simulink model "8Bit_Processor"  (R2019b)
settings: Solver=FixedStepDiscrete  StartTime=0.0  StopTime=10.0  RelTol=1e-3
libraries: hdlsllib x127, simulink_extras x9
(part 3 of 4)

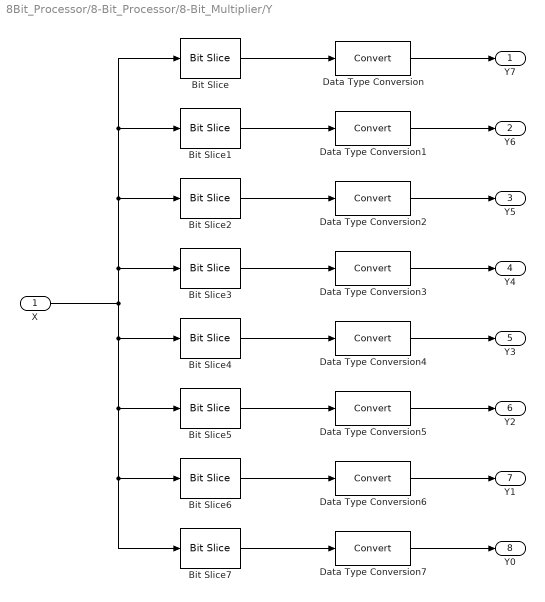
== system 8Bit_Processor/8-Bit_Processor/8-Bit_Multiplier/Y ==
  X : Inport  OutDataTypeStr=uint8  SampleTime=1
  Bit Slice : hdlsllib/Logic and Bit Operations/Bit Slice  lidx=7  ridx=7
      settings: SourceProductName=Simulink  SourceProductBaseCode=SL
  Bit Slice1 : hdlsllib/Logic and Bit Operations/Bit Slice  lidx=6  ridx=6
      settings: SourceProductName=Simulink  SourceProductBaseCode=SL
  Bit Slice2 : hdlsllib/Logic and Bit Operations/Bit Slice  lidx=5  ridx=5
      settings: SourceProductName=Simulink  SourceProductBaseCode=SL
  Bit Slice3 : hdlsllib/Logic and Bit Operations/Bit Slice  lidx=4  ridx=4
      settings: SourceProductName=Simulink  SourceProductBaseCode=SL
  Bit Slice4 : hdlsllib/Logic and Bit Operations/Bit Slice  lidx=3  ridx=3
      settings: SourceProductName=Simulink  SourceProductBaseCode=SL
  Bit Slice5 : hdlsllib/Logic and Bit Operations/Bit Slice  lidx=2  ridx=2
      settings: SourceProductName=Simulink  SourceProductBaseCode=SL
  Bit Slice6 : hdlsllib/Logic and Bit Operations/Bit Slice  lidx=1  ridx=1
      settings: SourceProductName=Simulink  SourceProductBaseCode=SL
  Bit Slice7 : hdlsllib/Logic and Bit Operations/Bit Slice  lidx=0  ridx=0
      settings: SourceProductName=Simulink  SourceProductBaseCode=SL
  Data Type Conversion{,1..7} (8 alike) : DataTypeConversion
  Y7 : Outport
  Y6 : Outport  Port=2
  Y5 : Outport  Port=3
  Y4 : Outport  Port=4
  Y3 : Outport  Port=5
  Y2 : Outport  Port=6
  Y1 : Outport  Port=7
  Y0 : Outport  Port=8
  wires:
  Bit Slice6/1 -> Data Type Conversion6/1
  X/1 -> Bit Slice3/1, Bit Slice2/1, Bit Slice1/1, Bit Slice/1, Bit Slice4/1, Bit Slice5/1, Bit Slice6/1, Bit Slice7/1
  Bit Slice/1 -> Data Type Conversion/1
  Bit Slice7/1 -> Data Type Conversion7/1
  Bit Slice4/1 -> Data Type Conversion4/1
  Bit Slice1/1 -> Data Type Conversion1/1
  Bit Slice3/1 -> Data Type Conversion3/1
  Data Type Conversion1/1 -> Y6/1
  Data Type Conversion7/1 -> Y0/1
  Data Type Conversion5/1 -> Y2/1
  Data Type Conversion3/1 -> Y4/1
  Data Type Conversion4/1 -> Y3/1
  Bit Slice2/1 -> Data Type Conversion2/1
  Bit Slice5/1 -> Data Type Conversion5/1
  Data Type Conversion6/1 -> Y1/1
  Data Type Conversion/1 -> Y7/1
  Data Type Conversion2/1 -> Y5/1

== system 8Bit_Processor/8-Bit_Processor/8-Bit_Register/Concat ==
  X0 : Inport  OutDataTypeStr=boolean  SampleTime=1
  X1 : Inport  Port=2  OutDataTypeStr=boolean  SampleTime=1
  X2 : Inport  Port=3  OutDataTypeStr=boolean  SampleTime=1
  X3 : Inport  Port=4  OutDataTypeStr=boolean  SampleTime=1
  X4 : Inport  Port=5  OutDataTypeStr=boolean  SampleTime=1
  X5 : Inport  Port=6  OutDataTypeStr=boolean  SampleTime=1
  X6 : Inport  Port=7  OutDataTypeStr=boolean  SampleTime=1
  X7 : Inport  Port=8  OutDataTypeStr=boolean  SampleTime=1
  Bit Concat : hdlsllib/Logic and Bit Operations/Bit Concat  numInputs=8
      settings: SourceProductName=Simulink
  Y : Outport  SampleTime=1
  wires:
  X6/1 -> Bit Concat/2
  X2/1 -> Bit Concat/6
  X7/1 -> Bit Concat/1
  X0/1 -> Bit Concat/8
  Bit Concat/1 -> Y/1
  X3/1 -> Bit Concat/5
  X1/1 -> Bit Concat/7
  X5/1 -> Bit Concat/3
  X4/1 -> Bit Concat/4

== system 8Bit_Processor/8-Bit_Processor/8-Bit_Register/Slicer ==
  X : Inport  OutDataTypeStr=uint8  SampleTime=1
  Bit Slice : hdlsllib/Logic and Bit Operations/Bit Slice  lidx=7  ridx=7
      settings: SourceProductName=Simulink  SourceProductBaseCode=SL
  Bit Slice1 : hdlsllib/Logic and Bit Operations/Bit Slice  lidx=6  ridx=6
      settings: SourceProductName=Simulink  SourceProductBaseCode=SL
  Bit Slice2 : hdlsllib/Logic and Bit Operations/Bit Slice  lidx=5  ridx=5
      settings: SourceProductName=Simulink  SourceProductBaseCode=SL
  Bit Slice3 : hdlsllib/Logic and Bit Operations/Bit Slice  lidx=4  ridx=4
      settings: SourceProductName=Simulink  SourceProductBaseCode=SL
  Bit Slice4 : hdlsllib/Logic and Bit Operations/Bit Slice  lidx=3  ridx=3
      settings: SourceProductName=Simulink  SourceProductBaseCode=SL
  Bit Slice5 : hdlsllib/Logic and Bit Operations/Bit Slice  lidx=2  ridx=2
      settings: SourceProductName=Simulink  SourceProductBaseCode=SL
  Bit Slice6 : hdlsllib/Logic and Bit Operations/Bit Slice  lidx=1  ridx=1
      settings: SourceProductName=Simulink  SourceProductBaseCode=SL
  Bit Slice7 : hdlsllib/Logic and Bit Operations/Bit Slice  lidx=0  ridx=0
      settings: SourceProductName=Simulink  SourceProductBaseCode=SL
  Data Type Conversion{,1..7} (8 alike) : DataTypeConversion  OutDataTypeStr=boolean
  Y7 : Outport  OutDataTypeStr=boolean  SampleTime=1
  Y6 : Outport  Port=2  OutDataTypeStr=boolean  SampleTime=1
  Y5 : Outport  Port=3  OutDataTypeStr=boolean  SampleTime=1
  Y4 : Outport  Port=4  OutDataTypeStr=boolean
  Y3 : Outport  Port=5  OutDataTypeStr=boolean  SampleTime=1
  Y2 : Outport  Port=6  OutDataTypeStr=boolean  SampleTime=1
  Y1 : Outport  Port=7  OutDataTypeStr=boolean  SampleTime=1
  Y0 : Outport  Port=8  OutDataTypeStr=boolean  SampleTime=1
  wires:
  Bit Slice6/1 -> Data Type Conversion6/1
  X/1 -> Bit Slice3/1, Bit Slice2/1, Bit Slice1/1, Bit Slice/1, Bit Slice4/1, Bit Slice5/1, Bit Slice6/1, Bit Slice7/1
  Bit Slice/1 -> Data Type Conversion/1
  Bit Slice7/1 -> Data Type Conversion7/1
  Bit Slice4/1 -> Data Type Conversion4/1
  Bit Slice1/1 -> Data Type Conversion1/1
  Bit Slice3/1 -> Data Type Conversion3/1
  Data Type Conversion1/1 -> Y6/1
  Data Type Conversion7/1 -> Y0/1
  Data Type Conversion5/1 -> Y2/1
  Data Type Conversion3/1 -> Y4/1
  Data Type Conversion4/1 -> Y3/1
  Bit Slice2/1 -> Data Type Conversion2/1
  Bit Slice5/1 -> Data Type Conversion5/1
  Data Type Conversion6/1 -> Y1/1
  Data Type Conversion/1 -> Y7/1
  Data Type Conversion2/1 -> Y5/1

== system 8Bit_Processor/8-Bit_Processor/8-Bit_Subtractor/Concat1 ==
  X7 : Inport  OutDataTypeStr=boolean  SampleTime=1
  X6 : Inport  Port=2  OutDataTypeStr=boolean  SampleTime=1
  X5 : Inport  Port=3  OutDataTypeStr=boolean  SampleTime=1
  X4 : Inport  Port=4  OutDataTypeStr=boolean  SampleTime=1
  X3 : Inport  Port=5  OutDataTypeStr=boolean  SampleTime=1
  X2 : Inport  Port=6  OutDataTypeStr=boolean  SampleTime=1
  X1 : Inport  Port=7  OutDataTypeStr=boolean  SampleTime=1
  X0 : Inport  Port=8  OutDataTypeStr=boolean  SampleTime=1
  Bit Concat : hdlsllib/Logic and Bit Operations/Bit Concat  numInputs=8
      settings: SourceProductName=Simulink
  Y : Outport
  wires:
  X6/1 -> Bit Concat/2
  X2/1 -> Bit Concat/6
  X7/1 -> Bit Concat/1
  X0/1 -> Bit Concat/8
  Bit Concat/1 -> Y/1
  X3/1 -> Bit Concat/5
  X1/1 -> Bit Concat/7
  X5/1 -> Bit Concat/3
  X4/1 -> Bit Concat/4

== system 8Bit_Processor/8-Bit_Processor/8-Bit_Subtractor/Full Subtractor ==
  In1 : Inport  OutDataTypeStr=boolean
  In2 : Inport  Port=2  OutDataTypeStr=boolean
  In3 : Inport  Port=3  OutDataTypeStr=boolean
  Half subtractor : Subsystem
  Half subtractor1 : Subsystem
  Logical Operator1 : Logic  Operator=OR  AllPortsSameDT=off  OutDataTypeStr=boolean
  Out1 : Outport
  Out2 : Outport  Port=2
  wires:
  Logical Operator1/1 -> Out2/1
  In1/1 -> Half subtractor/1(In1)
  Half subtractor1/1(Out1) -> Out1/1
  In2/1 -> Half subtractor/2(In2)
  In3/1 -> Half subtractor1/2(In2)
  Half subtractor/2(Out2) -> Logical Operator1/2
  Half subtractor/1(Out1) -> Half subtractor1/1(In1)
  Half subtractor1/2(Out2) -> Logical Operator1/1

== system 8Bit_Processor/8-Bit_Processor/8-Bit_Subtractor/Full Subtractor 2 ==
  In1 : Inport  OutDataTypeStr=boolean
  In2 : Inport  Port=2  OutDataTypeStr=boolean
  In3 : Inport  Port=3  OutDataTypeStr=boolean
  Half subtractor : Subsystem
  Half subtractor1 : Subsystem
  Logical Operator1 : Logic  Operator=OR  AllPortsSameDT=off  OutDataTypeStr=boolean
  Out1 : Outport
  Out2 : Outport  Port=2
  wires:
  Logical Operator1/1 -> Out2/1
  In1/1 -> Half subtractor/1(In1)
  Half subtractor1/1(Out1) -> Out1/1
  In2/1 -> Half subtractor/2(In2)
  In3/1 -> Half subtractor1/2(In2)
  Half subtractor/2(Out2) -> Logical Operator1/2
  Half subtractor/1(Out1) -> Half subtractor1/1(In1)
  Half subtractor1/2(Out2) -> Logical Operator1/1

== system 8Bit_Processor/8-Bit_Processor/8-Bit_Subtractor/Full Subtractor 3 ==
  In1 : Inport  OutDataTypeStr=boolean
  In2 : Inport  Port=2  OutDataTypeStr=boolean
  In3 : Inport  Port=3  OutDataTypeStr=boolean
  Half subtractor : Subsystem
  Half subtractor1 : Subsystem
  Logical Operator1 : Logic  Operator=OR  AllPortsSameDT=off  OutDataTypeStr=boolean
  Out1 : Outport
  Out2 : Outport  Port=2
  wires:
  Logical Operator1/1 -> Out2/1
  In1/1 -> Half subtractor/1(In1)
  Half subtractor1/1(Out1) -> Out1/1
  In2/1 -> Half subtractor/2(In2)
  In3/1 -> Half subtractor1/2(In2)
  Half subtractor/2(Out2) -> Logical Operator1/2
  Half subtractor/1(Out1) -> Half subtractor1/1(In1)
  Half subtractor1/2(Out2) -> Logical Operator1/1

== system 8Bit_Processor/8-Bit_Processor/8-Bit_Subtractor/Full Subtractor 4 ==
  In1 : Inport  OutDataTypeStr=boolean
  In2 : Inport  Port=2  OutDataTypeStr=boolean
  In3 : Inport  Port=3  OutDataTypeStr=boolean
  Half subtractor : Subsystem
  Half subtractor1 : Subsystem
  Logical Operator1 : Logic  Operator=OR  AllPortsSameDT=off  OutDataTypeStr=boolean
  Out1 : Outport
  Out2 : Outport  Port=2
  wires:
  Logical Operator1/1 -> Out2/1
  In1/1 -> Half subtractor/1(In1)
  Half subtractor1/1(Out1) -> Out1/1
  In2/1 -> Half subtractor/2(In2)
  In3/1 -> Half subtractor1/2(In2)
  Half subtractor/2(Out2) -> Logical Operator1/2
  Half subtractor/1(Out1) -> Half subtractor1/1(In1)
  Half subtractor1/2(Out2) -> Logical Operator1/1

== system 8Bit_Processor/8-Bit_Processor/8-Bit_Subtractor/Full Subtractor 5 ==
  In1 : Inport  OutDataTypeStr=boolean
  In2 : Inport  Port=2  OutDataTypeStr=boolean
  In3 : Inport  Port=3  OutDataTypeStr=boolean
  Half subtractor : Subsystem
  Half subtractor1 : Subsystem
  Logical Operator1 : Logic  Operator=OR  AllPortsSameDT=off  OutDataTypeStr=boolean
  Out1 : Outport
  Out2 : Outport  Port=2
  wires:
  Logical Operator1/1 -> Out2/1
  In1/1 -> Half subtractor/1(In1)
  Half subtractor1/1(Out1) -> Out1/1
  In2/1 -> Half subtractor/2(In2)
  In3/1 -> Half subtractor1/2(In2)
  Half subtractor/2(Out2) -> Logical Operator1/2
  Half subtractor/1(Out1) -> Half subtractor1/1(In1)
  Half subtractor1/2(Out2) -> Logical Operator1/1

== system 8Bit_Processor/8-Bit_Processor/8-Bit_Subtractor/Full Subtractor 6 ==
  In1 : Inport  OutDataTypeStr=boolean
  In2 : Inport  Port=2  OutDataTypeStr=boolean
  In3 : Inport  Port=3  OutDataTypeStr=boolean
  Half subtractor : Subsystem
  Half subtractor1 : Subsystem
  Logical Operator1 : Logic  Operator=OR  AllPortsSameDT=off  OutDataTypeStr=boolean
  Out1 : Outport
  Out2 : Outport  Port=2
  wires:
  Logical Operator1/1 -> Out2/1
  In1/1 -> Half subtractor/1(In1)
  Half subtractor1/1(Out1) -> Out1/1
  In2/1 -> Half subtractor/2(In2)
  In3/1 -> Half subtractor1/2(In2)
  Half subtractor/2(Out2) -> Logical Operator1/2
  Half subtractor/1(Out1) -> Half subtractor1/1(In1)
  Half subtractor1/2(Out2) -> Logical Operator1/1

== system 8Bit_Processor/8-Bit_Processor/8-Bit_Subtractor/Full Subtractor 7 ==
  In1 : Inport  OutDataTypeStr=boolean
  In2 : Inport  Port=2  OutDataTypeStr=boolean
  In3 : Inport  Port=3  OutDataTypeStr=boolean
  Half subtractor : Subsystem
  Half subtractor1 : Subsystem
  Logical Operator1 : Logic  Operator=OR  AllPortsSameDT=off  OutDataTypeStr=boolean
  Out1 : Outport
  Out2 : Outport  Port=2
  wires:
  Logical Operator1/1 -> Out2/1
  In1/1 -> Half subtractor/1(In1)
  Half subtractor1/1(Out1) -> Out1/1
  In2/1 -> Half subtractor/2(In2)
  In3/1 -> Half subtractor1/2(In2)
  Half subtractor/2(Out2) -> Logical Operator1/2
  Half subtractor/1(Out1) -> Half subtractor1/1(In1)
  Half subtractor1/2(Out2) -> Logical Operator1/1

== system 8Bit_Processor/8-Bit_Processor/8-Bit_Subtractor/Half subtractor ==
  In1 : Inport  OutDataTypeStr=boolean
  In2 : Inport  Port=2  OutDataTypeStr=boolean
  Logical Operator : Logic  AllPortsSameDT=off  OutDataTypeStr=boolean
  Logical Operator1 : Logic  Operator=XOR  AllPortsSameDT=off  OutDataTypeStr=boolean
  NOT : Logic  Operator=NOT  IconShape=distinctive  AllPortsSameDT=off  OutDataTypeStr=boolean
  Out1 : Outport
  Out2 : Outport  Port=2
  wires:
  In2/1 -> Logical Operator/2, Logical Operator1/2
  In1/1 -> NOT/1, Logical Operator1/1
  Logical Operator1/1 -> Out1/1
  Logical Operator/1 -> Out2/1
  NOT/1 -> Logical Operator/1

== system 8Bit_Processor/8-Bit_Processor/8-Bit_Subtractor/Slicer1 ==
  X : Inport  OutDataTypeStr=uint8  SampleTime=1
  Bit Slice : hdlsllib/Logic and Bit Operations/Bit Slice  lidx=7  ridx=7
      settings: SourceProductName=Simulink  SourceProductBaseCode=SL
  Bit Slice1 : hdlsllib/Logic and Bit Operations/Bit Slice  lidx=6  ridx=6
      settings: SourceProductName=Simulink  SourceProductBaseCode=SL
  Bit Slice2 : hdlsllib/Logic and Bit Operations/Bit Slice  lidx=5  ridx=5
      settings: SourceProductName=Simulink  SourceProductBaseCode=SL
  Bit Slice3 : hdlsllib/Logic and Bit Operations/Bit Slice  lidx=4  ridx=4
      settings: SourceProductName=Simulink  SourceProductBaseCode=SL
  Bit Slice4 : hdlsllib/Logic and Bit Operations/Bit Slice  lidx=3  ridx=3
      settings: SourceProductName=Simulink  SourceProductBaseCode=SL
  Bit Slice5 : hdlsllib/Logic and Bit Operations/Bit Slice  lidx=2  ridx=2
      settings: SourceProductName=Simulink  SourceProductBaseCode=SL
  Bit Slice6 : hdlsllib/Logic and Bit Operations/Bit Slice  lidx=1  ridx=1
      settings: SourceProductName=Simulink  SourceProductBaseCode=SL
  Bit Slice7 : hdlsllib/Logic and Bit Operations/Bit Slice  lidx=0  ridx=0
      settings: SourceProductName=Simulink  SourceProductBaseCode=SL
  Data Type Conversion{,1..7} (8 alike) : DataTypeConversion
  Y7 : Outport
  Y6 : Outport  Port=2
  Y5 : Outport  Port=3
  Y4 : Outport  Port=4
  Y3 : Outport  Port=5
  Y2 : Outport  Port=6
  Y1 : Outport  Port=7
  Y0 : Outport  Port=8
  wires:
  Bit Slice6/1 -> Data Type Conversion6/1
  X/1 -> Bit Slice3/1, Bit Slice2/1, Bit Slice1/1, Bit Slice/1, Bit Slice4/1, Bit Slice5/1, Bit Slice6/1, Bit Slice7/1
  Bit Slice/1 -> Data Type Conversion/1
  Bit Slice7/1 -> Data Type Conversion7/1
  Bit Slice4/1 -> Data Type Conversion4/1
  Bit Slice1/1 -> Data Type Conversion1/1
  Bit Slice3/1 -> Data Type Conversion3/1
  Data Type Conversion1/1 -> Y6/1
  Data Type Conversion7/1 -> Y0/1
  Data Type Conversion5/1 -> Y2/1
  Data Type Conversion3/1 -> Y4/1
  Data Type Conversion4/1 -> Y3/1
  Bit Slice2/1 -> Data Type Conversion2/1
  Bit Slice5/1 -> Data Type Conversion5/1
  Data Type Conversion6/1 -> Y1/1
  Data Type Conversion/1 -> Y7/1
  Data Type Conversion2/1 -> Y5/1

== system 8Bit_Processor/8-Bit_Processor/8-Bit_Subtractor/Slicer2 ==
  X : Inport  OutDataTypeStr=uint8  SampleTime=1
  Bit Slice : hdlsllib/Logic and Bit Operations/Bit Slice  lidx=7  ridx=7
      settings: SourceProductName=Simulink  SourceProductBaseCode=SL
  Bit Slice1 : hdlsllib/Logic and Bit Operations/Bit Slice  lidx=6  ridx=6
      settings: SourceProductName=Simulink  SourceProductBaseCode=SL
  Bit Slice2 : hdlsllib/Logic and Bit Operations/Bit Slice  lidx=5  ridx=5
      settings: SourceProductName=Simulink  SourceProductBaseCode=SL
  Bit Slice3 : hdlsllib/Logic and Bit Operations/Bit Slice  lidx=4  ridx=4
      settings: SourceProductName=Simulink  SourceProductBaseCode=SL
  Bit Slice4 : hdlsllib/Logic and Bit Operations/Bit Slice  lidx=3  ridx=3
      settings: SourceProductName=Simulink  SourceProductBaseCode=SL
  Bit Slice5 : hdlsllib/Logic and Bit Operations/Bit Slice  lidx=2  ridx=2
      settings: SourceProductName=Simulink  SourceProductBaseCode=SL
  Bit Slice6 : hdlsllib/Logic and Bit Operations/Bit Slice  lidx=1  ridx=1
      settings: SourceProductName=Simulink  SourceProductBaseCode=SL
  Bit Slice7 : hdlsllib/Logic and Bit Operations/Bit Slice  lidx=0  ridx=0
      settings: SourceProductName=Simulink  SourceProductBaseCode=SL
  Data Type Conversion{,1..7} (8 alike) : DataTypeConversion
  Y7 : Outport
  Y6 : Outport  Port=2
  Y5 : Outport  Port=3
  Y4 : Outport  Port=4
  Y3 : Outport  Port=5
  Y2 : Outport  Port=6
  Y1 : Outport  Port=7
  Y0 : Outport  Port=8
  wires:
  Bit Slice6/1 -> Data Type Conversion6/1
  X/1 -> Bit Slice3/1, Bit Slice2/1, Bit Slice1/1, Bit Slice/1, Bit Slice4/1, Bit Slice5/1, Bit Slice6/1, Bit Slice7/1
  Bit Slice/1 -> Data Type Conversion/1
  Bit Slice7/1 -> Data Type Conversion7/1
  Bit Slice4/1 -> Data Type Conversion4/1
  Bit Slice1/1 -> Data Type Conversion1/1
  Bit Slice3/1 -> Data Type Conversion3/1
  Data Type Conversion1/1 -> Y6/1
  Data Type Conversion7/1 -> Y0/1
  Data Type Conversion5/1 -> Y2/1
  Data Type Conversion3/1 -> Y4/1
  Data Type Conversion4/1 -> Y3/1
  Bit Slice2/1 -> Data Type Conversion2/1
  Bit Slice5/1 -> Data Type Conversion5/1
  Data Type Conversion6/1 -> Y1/1
  Data Type Conversion/1 -> Y7/1
  Data Type Conversion2/1 -> Y5/1

== system 8Bit_Processor/8-Bit_Processor/8-Bit 4-to-1 MUX/Subsystem/Slicer ==
  X : Inport  SampleTime=1
  Bit Slice6 : hdlsllib/Logic and Bit Operations/Bit Slice  lidx=1  ridx=1
      settings: SourceProductName=Simulink  SourceProductBaseCode=SL
  Bit Slice7 : hdlsllib/Logic and Bit Operations/Bit Slice  lidx=0  ridx=0
      settings: SourceProductName=Simulink  SourceProductBaseCode=SL
  Data Type Conversion6 : DataTypeConversion  OutDataTypeStr=boolean
  Data Type Conversion7 : DataTypeConversion  OutDataTypeStr=boolean
  A : Outport  OutDataTypeStr=boolean  SampleTime=1
  B : Outport  Port=2  OutDataTypeStr=boolean  SampleTime=1
  wires:
  Bit Slice6/1 -> Data Type Conversion6/1
  X/1 -> Bit Slice6/1, Bit Slice7/1
  Bit Slice7/1 -> Data Type Conversion7/1
  Data Type Conversion7/1 -> A/1
  Data Type Conversion6/1 -> B/1

== system 8Bit_Processor/8-Bit_Processor/8-Bit 4-to-1 MUX/Subsystem1/Slicer ==
  X : Inport  SampleTime=1
  Bit Slice6 : hdlsllib/Logic and Bit Operations/Bit Slice  lidx=1  ridx=1
      settings: SourceProductName=Simulink  SourceProductBaseCode=SL
  Bit Slice7 : hdlsllib/Logic and Bit Operations/Bit Slice  lidx=0  ridx=0
      settings: SourceProductName=Simulink  SourceProductBaseCode=SL
  Data Type Conversion6 : DataTypeConversion  OutDataTypeStr=boolean
  Data Type Conversion7 : DataTypeConversion  OutDataTypeStr=boolean
  A : Outport  OutDataTypeStr=boolean  SampleTime=1
  B : Outport  Port=2  OutDataTypeStr=boolean  SampleTime=1
  wires:
  Bit Slice6/1 -> Data Type Conversion6/1
  X/1 -> Bit Slice6/1, Bit Slice7/1
  Bit Slice7/1 -> Data Type Conversion7/1
  Data Type Conversion7/1 -> A/1
  Data Type Conversion6/1 -> B/1

== system 8Bit_Processor/8-Bit_Processor/8-Bit 4-to-1 MUX/Subsystem2/Slicer ==
  X : Inport  SampleTime=1
  Bit Slice6 : hdlsllib/Logic and Bit Operations/Bit Slice  lidx=1  ridx=1
      settings: SourceProductName=Simulink  SourceProductBaseCode=SL
  Bit Slice7 : hdlsllib/Logic and Bit Operations/Bit Slice  lidx=0  ridx=0
      settings: SourceProductName=Simulink  SourceProductBaseCode=SL
  Data Type Conversion6 : DataTypeConversion  OutDataTypeStr=boolean
  Data Type Conversion7 : DataTypeConversion  OutDataTypeStr=boolean
  A : Outport  OutDataTypeStr=boolean  SampleTime=1
  B : Outport  Port=2  OutDataTypeStr=boolean  SampleTime=1
  wires:
  Bit Slice6/1 -> Data Type Conversion6/1
  X/1 -> Bit Slice6/1, Bit Slice7/1
  Bit Slice7/1 -> Data Type Conversion7/1
  Data Type Conversion7/1 -> A/1
  Data Type Conversion6/1 -> B/1

== system 8Bit_Processor/8-Bit_Processor/8-Bit 4-to-1 MUX/Subsystem3/Slicer ==
  X : Inport  SampleTime=1
  Bit Slice6 : hdlsllib/Logic and Bit Operations/Bit Slice  lidx=1  ridx=1
      settings: SourceProductName=Simulink  SourceProductBaseCode=SL
  Bit Slice7 : hdlsllib/Logic and Bit Operations/Bit Slice  lidx=0  ridx=0
      settings: SourceProductName=Simulink  SourceProductBaseCode=SL
  Data Type Conversion6 : DataTypeConversion  OutDataTypeStr=boolean
  Data Type Conversion7 : DataTypeConversion  OutDataTypeStr=boolean
  A : Outport  OutDataTypeStr=boolean  SampleTime=1
  B : Outport  Port=2  OutDataTypeStr=boolean  SampleTime=1
  wires:
  Bit Slice6/1 -> Data Type Conversion6/1
  X/1 -> Bit Slice6/1, Bit Slice7/1
  Bit Slice7/1 -> Data Type Conversion7/1
  Data Type Conversion7/1 -> A/1
  Data Type Conversion6/1 -> B/1

== system 8Bit_Processor/8-Bit_Processor/8-Bit 4-to-1 MUX/Subsystem4/Slicer ==
  X : Inport  SampleTime=1
  Bit Slice6 : hdlsllib/Logic and Bit Operations/Bit Slice  lidx=1  ridx=1
      settings: SourceProductName=Simulink  SourceProductBaseCode=SL
  Bit Slice7 : hdlsllib/Logic and Bit Operations/Bit Slice  lidx=0  ridx=0
      settings: SourceProductName=Simulink  SourceProductBaseCode=SL
  Data Type Conversion6 : DataTypeConversion  OutDataTypeStr=boolean
  Data Type Conversion7 : DataTypeConversion  OutDataTypeStr=boolean
  A : Outport  OutDataTypeStr=boolean  SampleTime=1
  B : Outport  Port=2  OutDataTypeStr=boolean  SampleTime=1
  wires:
  Bit Slice6/1 -> Data Type Conversion6/1
  X/1 -> Bit Slice6/1, Bit Slice7/1
  Bit Slice7/1 -> Data Type Conversion7/1
  Data Type Conversion7/1 -> A/1
  Data Type Conversion6/1 -> B/1

== system 8Bit_Processor/8-Bit_Processor/8-Bit 4-to-1 MUX/Subsystem5/Slicer ==
  X : Inport  SampleTime=1
  Bit Slice6 : hdlsllib/Logic and Bit Operations/Bit Slice  lidx=1  ridx=1
      settings: SourceProductName=Simulink  SourceProductBaseCode=SL
  Bit Slice7 : hdlsllib/Logic and Bit Operations/Bit Slice  lidx=0  ridx=0
      settings: SourceProductName=Simulink  SourceProductBaseCode=SL
  Data Type Conversion6 : DataTypeConversion  OutDataTypeStr=boolean
  Data Type Conversion7 : DataTypeConversion  OutDataTypeStr=boolean
  A : Outport  OutDataTypeStr=boolean  SampleTime=1
  B : Outport  Port=2  OutDataTypeStr=boolean  SampleTime=1
  wires:
  Bit Slice6/1 -> Data Type Conversion6/1
  X/1 -> Bit Slice6/1, Bit Slice7/1
  Bit Slice7/1 -> Data Type Conversion7/1
  Data Type Conversion7/1 -> A/1
  Data Type Conversion6/1 -> B/1

== system 8Bit_Processor/8-Bit_Processor/8-Bit 4-to-1 MUX/Subsystem6/Slicer ==
  X : Inport  SampleTime=1
  Bit Slice6 : hdlsllib/Logic and Bit Operations/Bit Slice  lidx=1  ridx=1
      settings: SourceProductName=Simulink  SourceProductBaseCode=SL
  Bit Slice7 : hdlsllib/Logic and Bit Operations/Bit Slice  lidx=0  ridx=0
      settings: SourceProductName=Simulink  SourceProductBaseCode=SL
  Data Type Conversion6 : DataTypeConversion  OutDataTypeStr=boolean
  Data Type Conversion7 : DataTypeConversion  OutDataTypeStr=boolean
  A : Outport  OutDataTypeStr=boolean  SampleTime=1
  B : Outport  Port=2  OutDataTypeStr=boolean  SampleTime=1
  wires:
  Bit Slice6/1 -> Data Type Conversion6/1
  X/1 -> Bit Slice6/1, Bit Slice7/1
  Bit Slice7/1 -> Data Type Conversion7/1
  Data Type Conversion7/1 -> A/1
  Data Type Conversion6/1 -> B/1

== system 8Bit_Processor/8-Bit_Processor/8-Bit 4-to-1 MUX/Subsystem7/Slicer ==
  X : Inport  SampleTime=1
  Bit Slice6 : hdlsllib/Logic and Bit Operations/Bit Slice  lidx=1  ridx=1
      settings: SourceProductName=Simulink  SourceProductBaseCode=SL
  Bit Slice7 : hdlsllib/Logic and Bit Operations/Bit Slice  lidx=0  ridx=0
      settings: SourceProductName=Simulink  SourceProductBaseCode=SL
  Data Type Conversion6 : DataTypeConversion  OutDataTypeStr=boolean
  Data Type Conversion7 : DataTypeConversion  OutDataTypeStr=boolean
  A : Outport  OutDataTypeStr=boolean  SampleTime=1
  B : Outport  Port=2  OutDataTypeStr=boolean  SampleTime=1
  wires:
  Bit Slice6/1 -> Data Type Conversion6/1
  X/1 -> Bit Slice6/1, Bit Slice7/1
  Bit Slice7/1 -> Data Type Conversion7/1
  Data Type Conversion7/1 -> A/1
  Data Type Conversion6/1 -> B/1

== system 8Bit_Processor/8-Bit_Processor/8-Bit_Adder/Full adder1/Half adder1 ==
  In1 : Inport  OutDataTypeStr=boolean
  In2 : Inport  Port=2  OutDataTypeStr=boolean
  Logical Operator : Logic  AllPortsSameDT=off  OutDataTypeStr=boolean
  Logical Operator1 : Logic  Operator=XOR  AllPortsSameDT=off  OutDataTypeStr=boolean
  Out1 : Outport
  Out2 : Outport  Port=2
  wires:
  In2/1 -> Logical Operator/2, Logical Operator1/2
  In1/1 -> Logical Operator/1, Logical Operator1/1
  Logical Operator1/1 -> Out1/1
  Logical Operator/1 -> Out2/1

== system 8Bit_Processor/8-Bit_Processor/8-Bit_Adder/Full adder1/Half adder2 ==
  In1 : Inport  OutDataTypeStr=boolean
  In2 : Inport  Port=2  OutDataTypeStr=boolean
  Logical Operator : Logic  AllPortsSameDT=off  OutDataTypeStr=boolean
  Logical Operator1 : Logic  Operator=XOR  AllPortsSameDT=off  OutDataTypeStr=boolean
  Out1 : Outport
  Out2 : Outport  Port=2
  wires:
  In2/1 -> Logical Operator/2, Logical Operator1/2
  In1/1 -> Logical Operator/1, Logical Operator1/1
  Logical Operator1/1 -> Out1/1
  Logical Operator/1 -> Out2/1

== system 8Bit_Processor/8-Bit_Processor/8-Bit_Adder/Full adder2/Half adder1 ==
  In1 : Inport  OutDataTypeStr=boolean
  In2 : Inport  Port=2  OutDataTypeStr=boolean
  Logical Operator : Logic  AllPortsSameDT=off  OutDataTypeStr=boolean
  Logical Operator1 : Logic  Operator=XOR  AllPortsSameDT=off  OutDataTypeStr=boolean
  Out1 : Outport
  Out2 : Outport  Port=2
  wires:
  In2/1 -> Logical Operator/2, Logical Operator1/2
  In1/1 -> Logical Operator/1, Logical Operator1/1
  Logical Operator1/1 -> Out1/1
  Logical Operator/1 -> Out2/1

== system 8Bit_Processor/8-Bit_Processor/8-Bit_Adder/Full adder2/Half adder2 ==
  In1 : Inport  OutDataTypeStr=boolean
  In2 : Inport  Port=2  OutDataTypeStr=boolean
  Logical Operator : Logic  AllPortsSameDT=off  OutDataTypeStr=boolean
  Logical Operator1 : Logic  Operator=XOR  AllPortsSameDT=off  OutDataTypeStr=boolean
  Out1 : Outport
  Out2 : Outport  Port=2
  wires:
  In2/1 -> Logical Operator/2, Logical Operator1/2
  In1/1 -> Logical Operator/1, Logical Operator1/1
  Logical Operator1/1 -> Out1/1
  Logical Operator/1 -> Out2/1

== system 8Bit_Processor/8-Bit_Processor/8-Bit_Adder/Full adder3/Half adder1 ==
  In1 : Inport  OutDataTypeStr=boolean
  In2 : Inport  Port=2  OutDataTypeStr=boolean
  Logical Operator : Logic  AllPortsSameDT=off  OutDataTypeStr=boolean
  Logical Operator1 : Logic  Operator=XOR  AllPortsSameDT=off  OutDataTypeStr=boolean
  Out1 : Outport
  Out2 : Outport  Port=2
  wires:
  In2/1 -> Logical Operator/2, Logical Operator1/2
  In1/1 -> Logical Operator/1, Logical Operator1/1
  Logical Operator1/1 -> Out1/1
  Logical Operator/1 -> Out2/1

== system 8Bit_Processor/8-Bit_Processor/8-Bit_Adder/Full adder3/Half adder2 ==
  In1 : Inport  OutDataTypeStr=boolean
  In2 : Inport  Port=2  OutDataTypeStr=boolean
  Logical Operator : Logic  AllPortsSameDT=off  OutDataTypeStr=boolean
  Logical Operator1 : Logic  Operator=XOR  AllPortsSameDT=off  OutDataTypeStr=boolean
  Out1 : Outport
  Out2 : Outport  Port=2
  wires:
  In2/1 -> Logical Operator/2, Logical Operator1/2
  In1/1 -> Logical Operator/1, Logical Operator1/1
  Logical Operator1/1 -> Out1/1
  Logical Operator/1 -> Out2/1

== system 8Bit_Processor/8-Bit_Processor/8-Bit_Adder/Full adder4/Half adder1 ==
  In1 : Inport  OutDataTypeStr=boolean
  In2 : Inport  Port=2  OutDataTypeStr=boolean
  Logical Operator : Logic  AllPortsSameDT=off  OutDataTypeStr=boolean
  Logical Operator1 : Logic  Operator=XOR  AllPortsSameDT=off  OutDataTypeStr=boolean
  Out1 : Outport
  Out2 : Outport  Port=2
  wires:
  In2/1 -> Logical Operator/2, Logical Operator1/2
  In1/1 -> Logical Operator/1, Logical Operator1/1
  Logical Operator1/1 -> Out1/1
  Logical Operator/1 -> Out2/1

== system 8Bit_Processor/8-Bit_Processor/8-Bit_Adder/Full adder4/Half adder2 ==
  In1 : Inport  OutDataTypeStr=boolean
  In2 : Inport  Port=2  OutDataTypeStr=boolean
  Logical Operator : Logic  AllPortsSameDT=off  OutDataTypeStr=boolean
  Logical Operator1 : Logic  Operator=XOR  AllPortsSameDT=off  OutDataTypeStr=boolean
  Out1 : Outport
  Out2 : Outport  Port=2
  wires:
  In2/1 -> Logical Operator/2, Logical Operator1/2
  In1/1 -> Logical Operator/1, Logical Operator1/1
  Logical Operator1/1 -> Out1/1
  Logical Operator/1 -> Out2/1

== system 8Bit_Processor/8-Bit_Processor/8-Bit_Adder/Full adder5/Half adder1 ==
  In1 : Inport  OutDataTypeStr=boolean
  In2 : Inport  Port=2  OutDataTypeStr=boolean
  Logical Operator : Logic  AllPortsSameDT=off  OutDataTypeStr=boolean
  Logical Operator1 : Logic  Operator=XOR  AllPortsSameDT=off  OutDataTypeStr=boolean
  Out1 : Outport
  Out2 : Outport  Port=2
  wires:
  In2/1 -> Logical Operator/2, Logical Operator1/2
  In1/1 -> Logical Operator/1, Logical Operator1/1
  Logical Operator1/1 -> Out1/1
  Logical Operator/1 -> Out2/1

== system 8Bit_Processor/8-Bit_Processor/8-Bit_Adder/Full adder5/Half adder2 ==
  In1 : Inport  OutDataTypeStr=boolean
  In2 : Inport  Port=2  OutDataTypeStr=boolean
  Logical Operator : Logic  AllPortsSameDT=off  OutDataTypeStr=boolean
  Logical Operator1 : Logic  Operator=XOR  AllPortsSameDT=off  OutDataTypeStr=boolean
  Out1 : Outport
  Out2 : Outport  Port=2
  wires:
  In2/1 -> Logical Operator/2, Logical Operator1/2
  In1/1 -> Logical Operator/1, Logical Operator1/1
  Logical Operator1/1 -> Out1/1
  Logical Operator/1 -> Out2/1

== system 8Bit_Processor/8-Bit_Processor/8-Bit_Adder/Full adder6/Half adder1 ==
  In1 : Inport  OutDataTypeStr=boolean
  In2 : Inport  Port=2  OutDataTypeStr=boolean
  Logical Operator : Logic  AllPortsSameDT=off  OutDataTypeStr=boolean
  Logical Operator1 : Logic  Operator=XOR  AllPortsSameDT=off  OutDataTypeStr=boolean
  Out1 : Outport
  Out2 : Outport  Port=2
  wires:
  In2/1 -> Logical Operator/2, Logical Operator1/2
  In1/1 -> Logical Operator/1, Logical Operator1/1
  Logical Operator1/1 -> Out1/1
  Logical Operator/1 -> Out2/1

== system 8Bit_Processor/8-Bit_Processor/8-Bit_Adder/Full adder6/Half adder2 ==
  In1 : Inport  OutDataTypeStr=boolean
  In2 : Inport  Port=2  OutDataTypeStr=boolean
  Logical Operator : Logic  AllPortsSameDT=off  OutDataTypeStr=boolean
  Logical Operator1 : Logic  Operator=XOR  AllPortsSameDT=off  OutDataTypeStr=boolean
  Out1 : Outport
  Out2 : Outport  Port=2
  wires:
  In2/1 -> Logical Operator/2, Logical Operator1/2
  In1/1 -> Logical Operator/1, Logical Operator1/1
  Logical Operator1/1 -> Out1/1
  Logical Operator/1 -> Out2/1

== system 8Bit_Processor/8-Bit_Processor/8-Bit_Adder/Full adder7/Half adder1 ==
  In1 : Inport  OutDataTypeStr=boolean
  In2 : Inport  Port=2  OutDataTypeStr=boolean
  Logical Operator : Logic  AllPortsSameDT=off  OutDataTypeStr=boolean
  Logical Operator1 : Logic  Operator=XOR  AllPortsSameDT=off  OutDataTypeStr=boolean
  Out1 : Outport
  Out2 : Outport  Port=2
  wires:
  In2/1 -> Logical Operator/2, Logical Operator1/2
  In1/1 -> Logical Operator/1, Logical Operator1/1
  Logical Operator1/1 -> Out1/1
  Logical Operator/1 -> Out2/1

== system 8Bit_Processor/8-Bit_Processor/8-Bit_Adder/Full adder7/Half adder2 ==
  In1 : Inport  OutDataTypeStr=boolean
  In2 : Inport  Port=2  OutDataTypeStr=boolean
  Logical Operator : Logic  AllPortsSameDT=off  OutDataTypeStr=boolean
  Logical Operator1 : Logic  Operator=XOR  AllPortsSameDT=off  OutDataTypeStr=boolean
  Out1 : Outport
  Out2 : Outport  Port=2
  wires:
  In2/1 -> Logical Operator/2, Logical Operator1/2
  In1/1 -> Logical Operator/1, Logical Operator1/1
  Logical Operator1/1 -> Out1/1
  Logical Operator/1 -> Out2/1

== system 8Bit_Processor/8-Bit_Processor/8-Bit_Multiplier/Full adder1/Half adder1 ==
  In1 : Inport  OutDataTypeStr=boolean
  In2 : Inport  Port=2  OutDataTypeStr=boolean
  Logical Operator : Logic  AllPortsSameDT=off  OutDataTypeStr=boolean
  Logical Operator1 : Logic  Operator=XOR  AllPortsSameDT=off  OutDataTypeStr=boolean
  Out1 : Outport
  Out2 : Outport  Port=2
  wires:
  In2/1 -> Logical Operator/2, Logical Operator1/2
  In1/1 -> Logical Operator/1, Logical Operator1/1
  Logical Operator1/1 -> Out1/1
  Logical Operator/1 -> Out2/1

== system 8Bit_Processor/8-Bit_Processor/8-Bit_Multiplier/Full adder1/Half adder2 ==
  In1 : Inport  OutDataTypeStr=boolean
  In2 : Inport  Port=2  OutDataTypeStr=boolean
  Logical Operator : Logic  AllPortsSameDT=off  OutDataTypeStr=boolean
  Logical Operator1 : Logic  Operator=XOR  AllPortsSameDT=off  OutDataTypeStr=boolean
  Out1 : Outport
  Out2 : Outport  Port=2
  wires:
  In2/1 -> Logical Operator/2, Logical Operator1/2
  In1/1 -> Logical Operator/1, Logical Operator1/1
  Logical Operator1/1 -> Out1/1
  Logical Operator/1 -> Out2/1

== system 8Bit_Processor/8-Bit_Processor/8-Bit_Multiplier/Full adder10/Half adder1 ==
  In1 : Inport  OutDataTypeStr=boolean
  In2 : Inport  Port=2  OutDataTypeStr=boolean
  Logical Operator : Logic  AllPortsSameDT=off  OutDataTypeStr=boolean
  Logical Operator1 : Logic  Operator=XOR  AllPortsSameDT=off  OutDataTypeStr=boolean
  Out1 : Outport
  Out2 : Outport  Port=2
  wires:
  In2/1 -> Logical Operator/2, Logical Operator1/2
  In1/1 -> Logical Operator/1, Logical Operator1/1
  Logical Operator1/1 -> Out1/1
  Logical Operator/1 -> Out2/1

== system 8Bit_Processor/8-Bit_Processor/8-Bit_Multiplier/Full adder10/Half adder2 ==
  In1 : Inport  OutDataTypeStr=boolean
  In2 : Inport  Port=2  OutDataTypeStr=boolean
  Logical Operator : Logic  AllPortsSameDT=off  OutDataTypeStr=boolean
  Logical Operator1 : Logic  Operator=XOR  AllPortsSameDT=off  OutDataTypeStr=boolean
  Out1 : Outport
  Out2 : Outport  Port=2
  wires:
  In2/1 -> Logical Operator/2, Logical Operator1/2
  In1/1 -> Logical Operator/1, Logical Operator1/1
  Logical Operator1/1 -> Out1/1
  Logical Operator/1 -> Out2/1

== system 8Bit_Processor/8-Bit_Processor/8-Bit_Multiplier/Full adder11/Half adder1 ==
  In1 : Inport  OutDataTypeStr=boolean
  In2 : Inport  Port=2  OutDataTypeStr=boolean
  Logical Operator : Logic  AllPortsSameDT=off  OutDataTypeStr=boolean
  Logical Operator1 : Logic  Operator=XOR  AllPortsSameDT=off  OutDataTypeStr=boolean
  Out1 : Outport
  Out2 : Outport  Port=2
  wires:
  In2/1 -> Logical Operator/2, Logical Operator1/2
  In1/1 -> Logical Operator/1, Logical Operator1/1
  Logical Operator1/1 -> Out1/1
  Logical Operator/1 -> Out2/1

== system 8Bit_Processor/8-Bit_Processor/8-Bit_Multiplier/Full adder11/Half adder2 ==
  In1 : Inport  OutDataTypeStr=boolean
  In2 : Inport  Port=2  OutDataTypeStr=boolean
  Logical Operator : Logic  AllPortsSameDT=off  OutDataTypeStr=boolean
  Logical Operator1 : Logic  Operator=XOR  AllPortsSameDT=off  OutDataTypeStr=boolean
  Out1 : Outport
  Out2 : Outport  Port=2
  wires:
  In2/1 -> Logical Operator/2, Logical Operator1/2
  In1/1 -> Logical Operator/1, Logical Operator1/1
  Logical Operator1/1 -> Out1/1
  Logical Operator/1 -> Out2/1

== system 8Bit_Processor/8-Bit_Processor/8-Bit_Multiplier/Full adder12/Half adder1 ==
  In1 : Inport  OutDataTypeStr=boolean
  In2 : Inport  Port=2  OutDataTypeStr=boolean
  Logical Operator : Logic  AllPortsSameDT=off  OutDataTypeStr=boolean
  Logical Operator1 : Logic  Operator=XOR  AllPortsSameDT=off  OutDataTypeStr=boolean
  Out1 : Outport
  Out2 : Outport  Port=2
  wires:
  In2/1 -> Logical Operator/2, Logical Operator1/2
  In1/1 -> Logical Operator/1, Logical Operator1/1
  Logical Operator1/1 -> Out1/1
  Logical Operator/1 -> Out2/1

== system 8Bit_Processor/8-Bit_Processor/8-Bit_Multiplier/Full adder12/Half adder2 ==
  In1 : Inport  OutDataTypeStr=boolean
  In2 : Inport  Port=2  OutDataTypeStr=boolean
  Logical Operator : Logic  AllPortsSameDT=off  OutDataTypeStr=boolean
  Logical Operator1 : Logic  Operator=XOR  AllPortsSameDT=off  OutDataTypeStr=boolean
  Out1 : Outport
  Out2 : Outport  Port=2
  wires:
  In2/1 -> Logical Operator/2, Logical Operator1/2
  In1/1 -> Logical Operator/1, Logical Operator1/1
  Logical Operator1/1 -> Out1/1
  Logical Operator/1 -> Out2/1

== system 8Bit_Processor/8-Bit_Processor/8-Bit_Multiplier/Full adder13/Half adder1 ==
  In1 : Inport  OutDataTypeStr=boolean
  In2 : Inport  Port=2  OutDataTypeStr=boolean
  Logical Operator : Logic  AllPortsSameDT=off  OutDataTypeStr=boolean
  Logical Operator1 : Logic  Operator=XOR  AllPortsSameDT=off  OutDataTypeStr=boolean
  Out1 : Outport
  Out2 : Outport  Port=2
  wires:
  In2/1 -> Logical Operator/2, Logical Operator1/2
  In1/1 -> Logical Operator/1, Logical Operator1/1
  Logical Operator1/1 -> Out1/1
  Logical Operator/1 -> Out2/1

== system 8Bit_Processor/8-Bit_Processor/8-Bit_Multiplier/Full adder13/Half adder2 ==
  In1 : Inport  OutDataTypeStr=boolean
  In2 : Inport  Port=2  OutDataTypeStr=boolean
  Logical Operator : Logic  AllPortsSameDT=off  OutDataTypeStr=boolean
  Logical Operator1 : Logic  Operator=XOR  AllPortsSameDT=off  OutDataTypeStr=boolean
  Out1 : Outport
  Out2 : Outport  Port=2
  wires:
  In2/1 -> Logical Operator/2, Logical Operator1/2
  In1/1 -> Logical Operator/1, Logical Operator1/1
  Logical Operator1/1 -> Out1/1
  Logical Operator/1 -> Out2/1

== system 8Bit_Processor/8-Bit_Processor/8-Bit_Multiplier/Full adder14/Half adder1 ==
  In1 : Inport  OutDataTypeStr=boolean
  In2 : Inport  Port=2  OutDataTypeStr=boolean
  Logical Operator : Logic  AllPortsSameDT=off  OutDataTypeStr=boolean
  Logical Operator1 : Logic  Operator=XOR  AllPortsSameDT=off  OutDataTypeStr=boolean
  Out1 : Outport
  Out2 : Outport  Port=2
  wires:
  In2/1 -> Logical Operator/2, Logical Operator1/2
  In1/1 -> Logical Operator/1, Logical Operator1/1
  Logical Operator1/1 -> Out1/1
  Logical Operator/1 -> Out2/1

== system 8Bit_Processor/8-Bit_Processor/8-Bit_Multiplier/Full adder14/Half adder2 ==
  In1 : Inport  OutDataTypeStr=boolean
  In2 : Inport  Port=2  OutDataTypeStr=boolean
  Logical Operator : Logic  AllPortsSameDT=off  OutDataTypeStr=boolean
  Logical Operator1 : Logic  Operator=XOR  AllPortsSameDT=off  OutDataTypeStr=boolean
  Out1 : Outport
  Out2 : Outport  Port=2
  wires:
  In2/1 -> Logical Operator/2, Logical Operator1/2
  In1/1 -> Logical Operator/1, Logical Operator1/1
  Logical Operator1/1 -> Out1/1
  Logical Operator/1 -> Out2/1

== system 8Bit_Processor/8-Bit_Processor/8-Bit_Multiplier/Full adder15/Half adder1 ==
  In1 : Inport  OutDataTypeStr=boolean
  In2 : Inport  Port=2  OutDataTypeStr=boolean
  Logical Operator : Logic  AllPortsSameDT=off  OutDataTypeStr=boolean
  Logical Operator1 : Logic  Operator=XOR  AllPortsSameDT=off  OutDataTypeStr=boolean
  Out1 : Outport
  Out2 : Outport  Port=2
  wires:
  In2/1 -> Logical Operator/2, Logical Operator1/2
  In1/1 -> Logical Operator/1, Logical Operator1/1
  Logical Operator1/1 -> Out1/1
  Logical Operator/1 -> Out2/1

== system 8Bit_Processor/8-Bit_Processor/8-Bit_Multiplier/Full adder15/Half adder2 ==
  In1 : Inport  OutDataTypeStr=boolean
  In2 : Inport  Port=2  OutDataTypeStr=boolean
  Logical Operator : Logic  AllPortsSameDT=off  OutDataTypeStr=boolean
  Logical Operator1 : Logic  Operator=XOR  AllPortsSameDT=off  OutDataTypeStr=boolean
  Out1 : Outport
  Out2 : Outport  Port=2
  wires:
  In2/1 -> Logical Operator/2, Logical Operator1/2
  In1/1 -> Logical Operator/1, Logical Operator1/1
  Logical Operator1/1 -> Out1/1
  Logical Operator/1 -> Out2/1

== system 8Bit_Processor/8-Bit_Processor/8-Bit_Multiplier/Full adder16/Half adder1 ==
  In1 : Inport  OutDataTypeStr=boolean
  In2 : Inport  Port=2  OutDataTypeStr=boolean
  Logical Operator : Logic  AllPortsSameDT=off  OutDataTypeStr=boolean
  Logical Operator1 : Logic  Operator=XOR  AllPortsSameDT=off  OutDataTypeStr=boolean
  Out1 : Outport
  Out2 : Outport  Port=2
  wires:
  In2/1 -> Logical Operator/2, Logical Operator1/2
  In1/1 -> Logical Operator/1, Logical Operator1/1
  Logical Operator1/1 -> Out1/1
  Logical Operator/1 -> Out2/1

== system 8Bit_Processor/8-Bit_Processor/8-Bit_Multiplier/Full adder16/Half adder2 ==
  In1 : Inport  OutDataTypeStr=boolean
  In2 : Inport  Port=2  OutDataTypeStr=boolean
  Logical Operator : Logic  AllPortsSameDT=off  OutDataTypeStr=boolean
  Logical Operator1 : Logic  Operator=XOR  AllPortsSameDT=off  OutDataTypeStr=boolean
  Out1 : Outport
  Out2 : Outport  Port=2
  wires:
  In2/1 -> Logical Operator/2, Logical Operator1/2
  In1/1 -> Logical Operator/1, Logical Operator1/1
  Logical Operator1/1 -> Out1/1
  Logical Operator/1 -> Out2/1

== system 8Bit_Processor/8-Bit_Processor/8-Bit_Multiplier/Full adder17/Half adder1 ==
  In1 : Inport  OutDataTypeStr=boolean
  In2 : Inport  Port=2  OutDataTypeStr=boolean
  Logical Operator : Logic  AllPortsSameDT=off  OutDataTypeStr=boolean
  Logical Operator1 : Logic  Operator=XOR  AllPortsSameDT=off  OutDataTypeStr=boolean
  Out1 : Outport
  Out2 : Outport  Port=2
  wires:
  In2/1 -> Logical Operator/2, Logical Operator1/2
  In1/1 -> Logical Operator/1, Logical Operator1/1
  Logical Operator1/1 -> Out1/1
  Logical Operator/1 -> Out2/1

== system 8Bit_Processor/8-Bit_Processor/8-Bit_Multiplier/Full adder17/Half adder2 ==
  In1 : Inport  OutDataTypeStr=boolean
  In2 : Inport  Port=2  OutDataTypeStr=boolean
  Logical Operator : Logic  AllPortsSameDT=off  OutDataTypeStr=boolean
  Logical Operator1 : Logic  Operator=XOR  AllPortsSameDT=off  OutDataTypeStr=boolean
  Out1 : Outport
  Out2 : Outport  Port=2
  wires:
  In2/1 -> Logical Operator/2, Logical Operator1/2
  In1/1 -> Logical Operator/1, Logical Operator1/1
  Logical Operator1/1 -> Out1/1
  Logical Operator/1 -> Out2/1

== system 8Bit_Processor/8-Bit_Processor/8-Bit_Multiplier/Full adder18/Half adder1 ==
  In1 : Inport  OutDataTypeStr=boolean
  In2 : Inport  Port=2  OutDataTypeStr=boolean
  Logical Operator : Logic  AllPortsSameDT=off  OutDataTypeStr=boolean
  Logical Operator1 : Logic  Operator=XOR  AllPortsSameDT=off  OutDataTypeStr=boolean
  Out1 : Outport
  Out2 : Outport  Port=2
  wires:
  In2/1 -> Logical Operator/2, Logical Operator1/2
  In1/1 -> Logical Operator/1, Logical Operator1/1
  Logical Operator1/1 -> Out1/1
  Logical Operator/1 -> Out2/1

== system 8Bit_Processor/8-Bit_Processor/8-Bit_Multiplier/Full adder18/Half adder2 ==
  In1 : Inport  OutDataTypeStr=boolean
  In2 : Inport  Port=2  OutDataTypeStr=boolean
  Logical Operator : Logic  AllPortsSameDT=off  OutDataTypeStr=boolean
  Logical Operator1 : Logic  Operator=XOR  AllPortsSameDT=off  OutDataTypeStr=boolean
  Out1 : Outport
  Out2 : Outport  Port=2
  wires:
  In2/1 -> Logical Operator/2, Logical Operator1/2
  In1/1 -> Logical Operator/1, Logical Operator1/1
  Logical Operator1/1 -> Out1/1
  Logical Operator/1 -> Out2/1

== system 8Bit_Processor/8-Bit_Processor/8-Bit_Multiplier/Full adder19/Half adder1 ==
  In1 : Inport  OutDataTypeStr=boolean
  In2 : Inport  Port=2  OutDataTypeStr=boolean
  Logical Operator : Logic  AllPortsSameDT=off  OutDataTypeStr=boolean
  Logical Operator1 : Logic  Operator=XOR  AllPortsSameDT=off  OutDataTypeStr=boolean
  Out1 : Outport
  Out2 : Outport  Port=2
  wires:
  In2/1 -> Logical Operator/2, Logical Operator1/2
  In1/1 -> Logical Operator/1, Logical Operator1/1
  Logical Operator1/1 -> Out1/1
  Logical Operator/1 -> Out2/1

== system 8Bit_Processor/8-Bit_Processor/8-Bit_Multiplier/Full adder19/Half adder2 ==
  In1 : Inport  OutDataTypeStr=boolean
  In2 : Inport  Port=2  OutDataTypeStr=boolean
  Logical Operator : Logic  AllPortsSameDT=off  OutDataTypeStr=boolean
  Logical Operator1 : Logic  Operator=XOR  AllPortsSameDT=off  OutDataTypeStr=boolean
  Out1 : Outport
  Out2 : Outport  Port=2
  wires:
  In2/1 -> Logical Operator/2, Logical Operator1/2
  In1/1 -> Logical Operator/1, Logical Operator1/1
  Logical Operator1/1 -> Out1/1
  Logical Operator/1 -> Out2/1

== system 8Bit_Processor/8-Bit_Processor/8-Bit_Multiplier/Full adder2/Half adder1 ==
  In1 : Inport  OutDataTypeStr=boolean
  In2 : Inport  Port=2  OutDataTypeStr=boolean
  Logical Operator : Logic  AllPortsSameDT=off  OutDataTypeStr=boolean
  Logical Operator1 : Logic  Operator=XOR  AllPortsSameDT=off  OutDataTypeStr=boolean
  Out1 : Outport
  Out2 : Outport  Port=2
  wires:
  In2/1 -> Logical Operator/2, Logical Operator1/2
  In1/1 -> Logical Operator/1, Logical Operator1/1
  Logical Operator1/1 -> Out1/1
  Logical Operator/1 -> Out2/1

== system 8Bit_Processor/8-Bit_Processor/8-Bit_Multiplier/Full adder2/Half adder2 ==
  In1 : Inport  OutDataTypeStr=boolean
  In2 : Inport  Port=2  OutDataTypeStr=boolean
  Logical Operator : Logic  AllPortsSameDT=off  OutDataTypeStr=boolean
  Logical Operator1 : Logic  Operator=XOR  AllPortsSameDT=off  OutDataTypeStr=boolean
  Out1 : Outport
  Out2 : Outport  Port=2
  wires:
  In2/1 -> Logical Operator/2, Logical Operator1/2
  In1/1 -> Logical Operator/1, Logical Operator1/1
  Logical Operator1/1 -> Out1/1
  Logical Operator/1 -> Out2/1

== system 8Bit_Processor/8-Bit_Processor/8-Bit_Multiplier/Full adder20/Half adder1 ==
  In1 : Inport  OutDataTypeStr=boolean
  In2 : Inport  Port=2  OutDataTypeStr=boolean
  Logical Operator : Logic  AllPortsSameDT=off  OutDataTypeStr=boolean
  Logical Operator1 : Logic  Operator=XOR  AllPortsSameDT=off  OutDataTypeStr=boolean
  Out1 : Outport
  Out2 : Outport  Port=2
  wires:
  In2/1 -> Logical Operator/2, Logical Operator1/2
  In1/1 -> Logical Operator/1, Logical Operator1/1
  Logical Operator1/1 -> Out1/1
  Logical Operator/1 -> Out2/1

== system 8Bit_Processor/8-Bit_Processor/8-Bit_Multiplier/Full adder20/Half adder2 ==
  In1 : Inport  OutDataTypeStr=boolean
  In2 : Inport  Port=2  OutDataTypeStr=boolean
  Logical Operator : Logic  AllPortsSameDT=off  OutDataTypeStr=boolean
  Logical Operator1 : Logic  Operator=XOR  AllPortsSameDT=off  OutDataTypeStr=boolean
  Out1 : Outport
  Out2 : Outport  Port=2
  wires:
  In2/1 -> Logical Operator/2, Logical Operator1/2
  In1/1 -> Logical Operator/1, Logical Operator1/1
  Logical Operator1/1 -> Out1/1
  Logical Operator/1 -> Out2/1

== system 8Bit_Processor/8-Bit_Processor/8-Bit_Multiplier/Full adder21/Half adder1 ==
  In1 : Inport  OutDataTypeStr=boolean
  In2 : Inport  Port=2  OutDataTypeStr=boolean
  Logical Operator : Logic  AllPortsSameDT=off  OutDataTypeStr=boolean
  Logical Operator1 : Logic  Operator=XOR  AllPortsSameDT=off  OutDataTypeStr=boolean
  Out1 : Outport
  Out2 : Outport  Port=2
  wires:
  In2/1 -> Logical Operator/2, Logical Operator1/2
  In1/1 -> Logical Operator/1, Logical Operator1/1
  Logical Operator1/1 -> Out1/1
  Logical Operator/1 -> Out2/1

== system 8Bit_Processor/8-Bit_Processor/8-Bit_Multiplier/Full adder21/Half adder2 ==
  In1 : Inport  OutDataTypeStr=boolean
  In2 : Inport  Port=2  OutDataTypeStr=boolean
  Logical Operator : Logic  AllPortsSameDT=off  OutDataTypeStr=boolean
  Logical Operator1 : Logic  Operator=XOR  AllPortsSameDT=off  OutDataTypeStr=boolean
  Out1 : Outport
  Out2 : Outport  Port=2
  wires:
  In2/1 -> Logical Operator/2, Logical Operator1/2
  In1/1 -> Logical Operator/1, Logical Operator1/1
  Logical Operator1/1 -> Out1/1
  Logical Operator/1 -> Out2/1

== system 8Bit_Processor/8-Bit_Processor/8-Bit_Multiplier/Full adder22/Half adder1 ==
  In1 : Inport  OutDataTypeStr=boolean
  In2 : Inport  Port=2  OutDataTypeStr=boolean
  Logical Operator : Logic  AllPortsSameDT=off  OutDataTypeStr=boolean
  Logical Operator1 : Logic  Operator=XOR  AllPortsSameDT=off  OutDataTypeStr=boolean
  Out1 : Outport
  Out2 : Outport  Port=2
  wires:
  In2/1 -> Logical Operator/2, Logical Operator1/2
  In1/1 -> Logical Operator/1, Logical Operator1/1
  Logical Operator1/1 -> Out1/1
  Logical Operator/1 -> Out2/1

== system 8Bit_Processor/8-Bit_Processor/8-Bit_Multiplier/Full adder22/Half adder2 ==
  In1 : Inport  OutDataTypeStr=boolean
  In2 : Inport  Port=2  OutDataTypeStr=boolean
  Logical Operator : Logic  AllPortsSameDT=off  OutDataTypeStr=boolean
  Logical Operator1 : Logic  Operator=XOR  AllPortsSameDT=off  OutDataTypeStr=boolean
  Out1 : Outport
  Out2 : Outport  Port=2
  wires:
  In2/1 -> Logical Operator/2, Logical Operator1/2
  In1/1 -> Logical Operator/1, Logical Operator1/1
  Logical Operator1/1 -> Out1/1
  Logical Operator/1 -> Out2/1

== system 8Bit_Processor/8-Bit_Processor/8-Bit_Multiplier/Full adder23/Half adder1 ==
  In1 : Inport  OutDataTypeStr=boolean
  In2 : Inport  Port=2  OutDataTypeStr=boolean
  Logical Operator : Logic  AllPortsSameDT=off  OutDataTypeStr=boolean
  Logical Operator1 : Logic  Operator=XOR  AllPortsSameDT=off  OutDataTypeStr=boolean
  Out1 : Outport
  Out2 : Outport  Port=2
  wires:
  In2/1 -> Logical Operator/2, Logical Operator1/2
  In1/1 -> Logical Operator/1, Logical Operator1/1
  Logical Operator1/1 -> Out1/1
  Logical Operator/1 -> Out2/1

== system 8Bit_Processor/8-Bit_Processor/8-Bit_Multiplier/Full adder23/Half adder2 ==
  In1 : Inport  OutDataTypeStr=boolean
  In2 : Inport  Port=2  OutDataTypeStr=boolean
  Logical Operator : Logic  AllPortsSameDT=off  OutDataTypeStr=boolean
  Logical Operator1 : Logic  Operator=XOR  AllPortsSameDT=off  OutDataTypeStr=boolean
  Out1 : Outport
  Out2 : Outport  Port=2
  wires:
  In2/1 -> Logical Operator/2, Logical Operator1/2
  In1/1 -> Logical Operator/1, Logical Operator1/1
  Logical Operator1/1 -> Out1/1
  Logical Operator/1 -> Out2/1

== system 8Bit_Processor/8-Bit_Processor/8-Bit_Multiplier/Full adder24/Half adder1 ==
  In1 : Inport  OutDataTypeStr=boolean
  In2 : Inport  Port=2  OutDataTypeStr=boolean
  Logical Operator : Logic  AllPortsSameDT=off  OutDataTypeStr=boolean
  Logical Operator1 : Logic  Operator=XOR  AllPortsSameDT=off  OutDataTypeStr=boolean
  Out1 : Outport
  Out2 : Outport  Port=2
  wires:
  In2/1 -> Logical Operator/2, Logical Operator1/2
  In1/1 -> Logical Operator/1, Logical Operator1/1
  Logical Operator1/1 -> Out1/1
  Logical Operator/1 -> Out2/1

== system 8Bit_Processor/8-Bit_Processor/8-Bit_Multiplier/Full adder24/Half adder2 ==
  In1 : Inport  OutDataTypeStr=boolean
  In2 : Inport  Port=2  OutDataTypeStr=boolean
  Logical Operator : Logic  AllPortsSameDT=off  OutDataTypeStr=boolean
  Logical Operator1 : Logic  Operator=XOR  AllPortsSameDT=off  OutDataTypeStr=boolean
  Out1 : Outport
  Out2 : Outport  Port=2
  wires:
  In2/1 -> Logical Operator/2, Logical Operator1/2
  In1/1 -> Logical Operator/1, Logical Operator1/1
  Logical Operator1/1 -> Out1/1
  Logical Operator/1 -> Out2/1
